simulink model "plant_model"  (R2023b)
settings: Solver=VariableStepAuto  StartTime=0.0  StopTime=10.0  RelTol=1e-3
InitFcn:
  | Tstall = 20;
  | NoLoadSpeed = 20;
  | J_inertia = 1;
  | b_damping = 0;
  | load('MyTest.mat')
  | Vn = 30;
  | wNL = NoLoadSpeed;
  | K = Vn/wNL;
  | R = Vn^2/wNL/Tstall;
  | L = 1e-5;
model workspace (MAT data in the model file):
  plant_model_spesession : sldodialogs.data.SessionData (value not decoded)
undefined symbols (not defined in the file or in its folder): sigbuilder_block
settings Model: Creator=Harish  LastModifiedBy=Harish

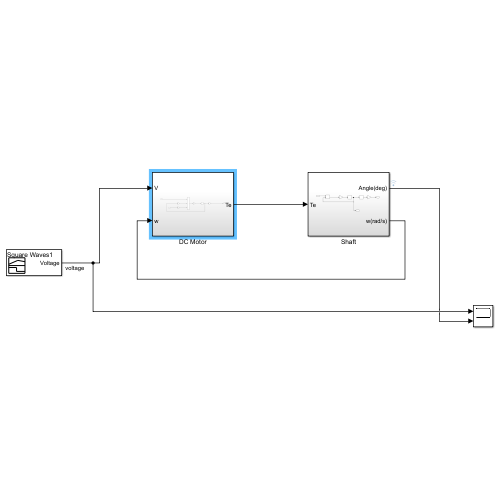
[thumbnail: Simulink's stored preview of the top-level diagram]
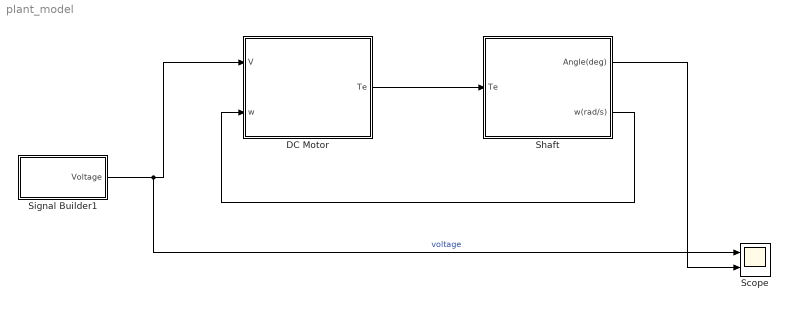
== system plant_model ==
  DC Motor : Subsystem
  Scope : Scope  NumInputPorts=2
  Shaft : Subsystem
  Signal Builder1 : Subsystem  Tag=STV Subsys  LoadFcn=sigbuilder_block('load');  StartFcn=sigbuilder_block('start');  StopFcn=sigbuilder_block('stop');  ClipboardFcn=sigbuilder_block('clipboard');  mask(Sigbuilder block){tuvar=[0:10]}
      mask help: Sigbuilder GUI
      mask init:
      | if ~strcmp(get_param(bdroot(gcbh),'SimulationStatus'),'stopped') tuvar = sigbuilder_block('maskInit'); end
      settings: CopyFcn=sigbuilder_block('copy');  DeleteFcn=sigbuilder_block('delete');  ModelCloseFcn=sigbuilder_block('modelClose');  PreSaveFcn=sigbuilder_block('preSave');  PauseFcn=sigbuilder_block('pause')  ContinueFcn=sigbuilder_block('continue')  NameChangeFcn=sigbuilder_block('namechange');  OpenFcn=sigbuilder_block('open',[495.75 237 550.5 399.75 ]);  CloseFcn=sigbuilder_block('close');
      mask Display: plot(0, 0, 100, 100,[2, 2, 32, 32, 2], [68, 8, 8, 68, 68],[32, 2], [38, 38], [32, 19, 2],[53, 60, 44], [32, 17, 17, 2],[16, 16, 31, 31]);txt = getActiveGroup(gcbh);text(2, 100, txt,'verticalAlignment', 'top');
  wires:
  DC Motor/1(Te) -> Shaft/1(Te)
  Shaft/2(w(rad/s)) -> DC Motor/2(w)
  Signal Builder1/1(Voltage) -> DC Motor/1(V), Scope/1  "voltage"
  Shaft/1(Angle(deg)) -> Scope/2

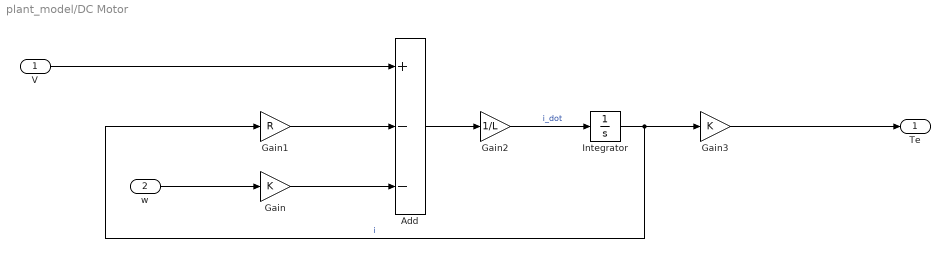
== system plant_model/DC Motor ==
  V : Inport
  w : Inport  Port=2
  Add : Sum  Inputs=+--
  Gain : Gain  Gain=K
  Gain1 : Gain  Gain=R
  Gain2 : Gain  Gain=1/L
  Gain3 : Gain  Gain=K
  Integrator : Integrator
  Te : Outport
  wires:
  V/1 -> Add/1
  Gain3/1 -> Te/1
  Gain1/1 -> Add/2
  Gain2/1 -> Integrator/1  "i_dot"
  Gain/1 -> Add/3
  Add/1 -> Gain2/1
  Integrator/1 -> Gain1/1, Gain3/1  "i"
  w/1 -> Gain/1

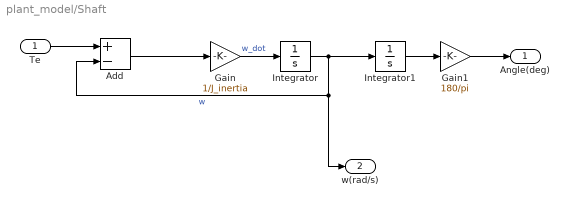
== system plant_model/Shaft ==
  Te : Inport
  Add : Sum  Inputs=+-
  Gain : Gain  Gain=1/J_inertia
  Gain1 : Gain  Gain=180/pi
  Integrator : Integrator
  Integrator1 : Integrator
  Angle(deg) : Outport
  w(rad/s) : Outport  Port=2
  wires:
  Te/1 -> Add/1
  Gain/1 -> Integrator/1  "w_dot"
  Integrator/1 -> Integrator1/1, Add/2, w(rad/s)/1  "w"
  Integrator1/1 -> Gain1/1
  Gain1/1 -> Angle(deg)/1
  Add/1 -> Gain/1

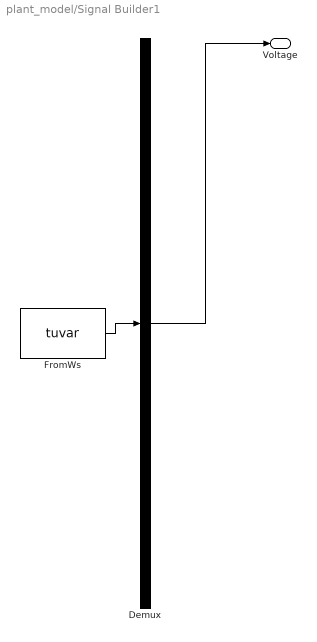
== system plant_model/Signal Builder1 ==
  Demux : Demux  Tag=STV Demux  Outputs=1
      settings: DisplayOption=none
  FromWs : FromWorkspace  Tag=STV FromWs  VariableName=tuvar  SampleTime=1/100
      SigBuilderData=|
      | common.afterFinalStr = 'Extrapolate'
      | common.sampleTime = '1/100'
      | dataSet(1).timeRange = [0 10]
      | dataSet(1).name = 'Bounds'
      | dataSet(2).timeRange = [0 10]
      | dataSet(2).name = 'Steps'
      | dataSet(3).timeRange = [0 10]
      | dataSet(3).name = 'Small Steps'
      | dataSet(4).timeRange = [0 10]
      | dataSet(4).name = 'Square Waves'
      | dataSet(5).timeRange = [0 10]
      | dataSet(5).name = 'Square Waves1'
      | sbobj.Groups(1).Name = 'Bounds'
      | sbobj.Groups(1).Signals.Name = 'Voltage'
      | sbobj.Groups(1).Signals.XData = [0 2 2 2.5 2.5 4.5 4.5 10]
      | sbobj.Groups(1).Signals.YData = [0 0 5 5 0 0 -5 -5]
      | sbobj.Groups(2).Name = 'Steps'
      | sbobj.Groups(2).Signals.Name = 'Voltage'
      | sbobj.Groups(2).Signals.XData = [0 1.52 1.52 2.4 2.4 3.66 3.68 4.64 4.64 6.02 6.02 7 7 8.96 8.96 10]
      | sbobj.Groups(2).Signals.YData = [2 2 -3 -3 3 -1 1.95 1.95 -2 -2 0.7 0.7 -1.05 -0.05 0 0]
      | sbobj.Groups(3).Name = 'Small Steps'
      | sbobj.Groups(3).Signals.Name = 'Voltage'
      | sbobj.Groups(3).Signals.XData = [0 0.5 0.5 1.02 1.02 2 2 2.58 2.58 3.78 3.78 4.64 4.64 5.28 5.28 6 6 7 7 9 9 10]
      | sbobj.Groups(3).Signals.YData = [0.4 0.4 0.75 0.75 1.5 3 1.55 1.55 3.55 3.55 -3.05 -3.05 -1 -1 -0.45 -0.45 0.7 0.7 -2.05 -0.05 1 1]
      | sbobj.Groups(4).Name = 'Square Waves'
      | sbobj.Groups(4).Signals.Name = 'Voltage'
      | sbobj.Groups(4).Signals.XData = [0 0.5 0.5 1.02 1.02 1.5 1.5 2 2 2.5 2.5 3 3 4 4 5 5 6 6 7 7 8 8 9 9 9.8 9.8 10]
      | sbobj.Groups(4).Signals.YData = [0.4 0.4 -0.4 -0.4 1 1 -1 -1 1.5 1.5 -1.5 -1.5 2 2 -2 -2 3 3 -3 -3 1.3 1.3 -1.3 -1.3 -4 -4 0 0]
      | sbobj.Groups(5).Name = 'Square Waves1'
      | sbobj.Groups(5).Signals.Name = 'Voltage'
      | sbobj.Groups(5).Signals.XData = [0 1 1 2 2 3 3 4 4 5 5 6 6 7 7 8 8 9 9 9.8 9.8 10]
      | sbobj.Groups(5).Signals.YData = [0 0.75 0 -0.75 0 1.5 0 -1.5 2 2 -2 -2 3 3 -3 -3 1 1 -1 -1 0 0]
  Voltage : Outport  Tag=STV Outport  VectorParamsAs1DForOutWhenUnconnected=off
  wires:
  Demux/1 -> Voltage/1
  FromWs/1 -> Demux/1
